simulink model "ECM_EKF_WLTP"  (R2021b)
settings: Solver=FixedStepDiscrete  StartTime=0.0  StopTime=10000  FixedStep=Ts_data  RelTol=1e-3
PreLoadFcn:
  | bdclose all
  | open_system('mdl/ECM_EKF_WLTP')
  | get_param(bdroot,'DataDictionary')
undefined symbols (not defined in the file or in its folder): C1_lut, C2_lut, crate_bp, DiscIntNeverNeededParam, R0_lut, R1_lut, R2_lut, raptor_get_param_eval, raptor_xcp_function, SoC0_guess, soc_bp, Ts_data
libraries: arc_dd_lib x12, Raptor_lib x8, arc_specialized_lib x4, simulink x2, arc_logic_lib x2, arc_fault_lib x2
(part 1 of 2)
settings Model: DataDictionary=ecm_dd.sldd  Creator=ahmeds28  LastModifiedBy=ahmeds28

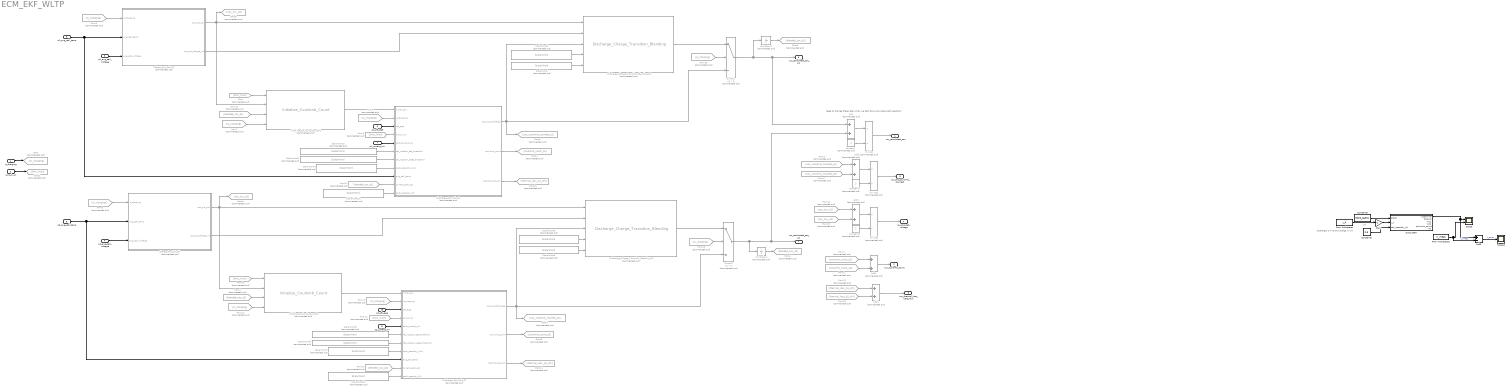
== system ECM_EKF_WLTP ==
  note: Need to change these later when we start allowing single pack operation
  note: discharge is +ve and charge is -ve
  is_charging : Inport  OutDataTypeStr=boolean
  bms_hvon : Inport  Port=2  OutDataTypeStr=boolean
  p1_avg_cell_voltage : Inport  Port=3  OutDataTypeStr=double
  p2_avg_cell_voltage : Inport  Port=4  OutDataTypeStr=double
  p1_avg_cell_temp : Inport  Port=5  OutDataTypeStr=double
  p2_avg_cell_temp : Inport  Port=6  OutDataTypeStr=double
  p1_current_mA : Inport  Port=7  OutDataTypeStr=double
  p2_current_mA : Inport  Port=8  OutDataTypeStr=double
  p1_sfp_age : Inport  Port=9  OutDataTypeStr=uint16
  p2_sfp_age : Inport  Port=10  OutDataTypeStr=uint16
  Add{,1..4} (5 alike) : Sum  Commented=on
  Add5 : Sum  Inputs=+-
  Charge_Soc_Calc_P1 : Subsystem  Commented=on
  Charge_Soc_Calc_P2 : Subsystem  Commented=on
  Constant : Constant  Commented=on  Value=2
  Constant1 : Constant  Commented=on  Value=2
  Constant2 : Constant  Commented=on  Value=2
  Constant3 : Constant  Value=2.5
  Constant5 : Constant  Value=SoC0_guess
  Discharge_Charge_Transition_Blending_P1 : arc_specialized_lib/Discharge_Charge_Transition_Blending  Commented=on  SystemSampleTime=-1  SSRTWFcnClass=[]  VariantActivationTime=update diagram  Latency=0  AutoFrameSizeCalculation=off
  Discharge_Charge_Transition_Blending_P2 : arc_specialized_lib/Discharge_Charge_Transition_Blending  Commented=on  SystemSampleTime=-1  SSRTWFcnClass=[]  VariantActivationTime=update diagram  Latency=0  AutoFrameSizeCalculation=off
  Discharge_Soc_Calc_P1 : Subsystem  Commented=on
  Discharge_Soc_Calc_P2 : Subsystem  Commented=on
  Divide : Product  Commented=on  Inputs=*/
  Divide1 : Product  Commented=on  Inputs=*/
  Divide2 : Product  Commented=on  Inputs=*/
  From{,9..10,12} (4 alike) : From  Commented=on  GotoTag=bms_hvon
  From Workspace : FromWorkspace  VariableName=I_A
  From Workspace1 : FromWorkspace  VariableName=V_meas
  From1 : From  Commented=on  GotoTag=coulomb_count_p1
  From{5..8,11,13,15..16} (8 alike) : From  Commented=on  GotoTag=is_charging
  From14 : From  Commented=on  GotoTag=blended_soc_p1
  From17 : From  Commented=on  GotoTag=soc_coulomb_counted_p2
  From18 : From  Commented=on  GotoTag=soc_ocv_p1
  From19 : From  Commented=on  GotoTag=soc_ocv_p2
  From2 : From  Commented=on  GotoTag=coulomb_count_p2
  From20 : From  Commented=on  GotoTag=blended_soc_p2
  From21 : From  Commented=on  GotoTag=blended_soc_p1
  From22 : From  Commented=on  GotoTag=thermal_loss_p1_Wh
  From23 : From  Commented=on  GotoTag=thermal_loss_p2_Wh
  From3 : From  Commented=on  GotoTag=soc_coulomb_counted_p1
  From4 : From  Commented=on  GotoTag=blended_soc_p2
  Gain : Gain  Gain=-1
  Goto : Goto  Commented=on  GotoTag=is_charging
  Goto1 : Goto  Commented=on  GotoTag=blended_soc_p2
  Goto10 : Goto  Commented=on  GotoTag=thermal_loss_p1_Wh
  Goto11 : Goto  Commented=on  GotoTag=thermal_loss_p2_Wh
  Goto2 : Goto  Commented=on  GotoTag=bms_hvon
  Goto3 : Goto  Commented=on  GotoTag=blended_soc_p1
  Goto4 : Goto  Commented=on  GotoTag=coulomb_count_p1
  Goto5 : Goto  Commented=on  GotoTag=coulomb_count_p2
  Goto6 : Goto  Commented=on  GotoTag=soc_coulomb_counted_p1
  Goto7 : Goto  Commented=on  GotoTag=soc_coulomb_counted_p2
  Goto8 : Goto  Commented=on  GotoTag=soc_ocv_p1
  Goto9 : Goto  Commented=on  GotoTag=soc_ocv_p2
  Initialize_Coulomb_Count_P1 : arc_specialized_lib/Initialize_Coulomb_Count  Commented=on  SystemSampleTime=-1  SSRTWFcnClass=[]  VariantActivationTime=update diagram  Latency=0  AutoFrameSizeCalculation=off
  Initialize_Coulomb_Count_P2 : arc_specialized_lib/Initialize_Coulomb_Count  Commented=on  SystemSampleTime=-1  SSRTWFcnClass=[]  VariantActivationTime=update diagram  Latency=0  AutoFrameSizeCalculation=off
  ScalarWord : arc_dd_lib/DataParam/ScalarWord  Tag=TYPE:UInt8; LSB:0.015625; OFF:0; RANGE:(0,3); UNIT:adm;  Description=Scalar Calibration  Commented=on  ScalarVar_Name=charge_soc_upper_limit  ScalarVar_Value=95  ScalarVar_Min=0  ScalarVar_Max=100  ScalarVar_dType=uint8  ScalarVar_dUnit=%  ScalarVar_dT=inf  ScalarVar_vType=Coefficient (k)  ScalarVar_Description=Insert variable description here.  SSRTWFcnClass=[]
  ScalarWord1 : arc_dd_lib/DataParam/ScalarWord  Tag=TYPE:UInt8; LSB:0.015625; OFF:0; RANGE:(0,3); UNIT:adm;  Description=Scalar Calibration  Commented=on  ScalarVar_Name=blending_distance  ScalarVar_Value=20  ScalarVar_Min=0  ScalarVar_Max=100  ScalarVar_dType=uint8  ScalarVar_dUnit=%  ScalarVar_dT=inf  ScalarVar_vType=Coefficient (k)  ScalarVar_Description=Insert variable description here.  SSRTWFcnClass=[]
  ScalarWord10 : arc_dd_lib/DataParam/ScalarWord  Tag=TYPE:UInt8; LSB:0.015625; OFF:0; RANGE:(0,3); UNIT:adm;  Description=Scalar Calibration  Commented=on  ScalarVar_Name=single_pack_energy_capacity  ScalarVar_Value=110000  ScalarVar_Min=0  ScalarVar_Max=1e7  ScalarVar_dType=uint32  ScalarVar_dUnit=Wh  ScalarVar_dT=inf  ScalarVar_vType=Coefficient (k)  ScalarVar_Description=Insert variable description here.  SSRTWFcnClass=[]
  ScalarWord11 : arc_dd_lib/DataParam/ScalarWord  Tag=TYPE:UInt8; LSB:0.015625; OFF:0; RANGE:(0,3); UNIT:adm;  Description=Scalar Calibration  Commented=on  ScalarVar_Name=single_pack_energy_capacity  ScalarVar_Value=110000  ScalarVar_Min=0  ScalarVar_Max=1e7  ScalarVar_dType=uint32  ScalarVar_dUnit=Wh  ScalarVar_dT=inf  ScalarVar_vType=Coefficient (k)  ScalarVar_Description=Insert variable description here.  SSRTWFcnClass=[]
  ScalarWord2 : arc_dd_lib/DataParam/ScalarWord  Tag=TYPE:UInt8; LSB:0.015625; OFF:0; RANGE:(0,3); UNIT:adm;  Description=Scalar Calibration  Commented=on  ScalarVar_Name=current_sensor_lossCan_set_threshold  ScalarVar_Value=100  ScalarVar_Min=0  ScalarVar_Max=65534  ScalarVar_dType=uint16  ScalarVar_dT=inf  ScalarVar_vType=Coefficient (k)  ScalarVar_Description=Insert variable description here.  SSRTWFcnClass=[]
  ScalarWord3 : arc_dd_lib/DataParam/ScalarWord  Tag=TYPE:UInt8; LSB:0.015625; OFF:0; RANGE:(0,3); UNIT:adm;  Description=Scalar Calibration  Commented=on  ScalarVar_Name=current_sensor_lossCan_reset_threshold  ScalarVar_Value=0  ScalarVar_Min=0  ScalarVar_Max=65534  ScalarVar_dType=uint16  ScalarVar_dT=inf  ScalarVar_vType=Coefficient (k)  ScalarVar_Description=Insert variable description here.  SSRTWFcnClass=[]
  ScalarWord4 : arc_dd_lib/DataParam/ScalarWord  Tag=TYPE:UInt8; LSB:0.015625; OFF:0; RANGE:(0,3); UNIT:adm;  Description=Scalar Calibration  Commented=on  ScalarVar_Name=single_pack_capacity  ScalarVar_Value=160000  ScalarVar_Min=0  ScalarVar_Max=1e7  ScalarVar_dType=uint32  ScalarVar_dUnit=mAh  ScalarVar_dT=inf  ScalarVar_vType=Coefficient (k)  ScalarVar_Description=Insert variable description here.  SSRTWFcnClass=[]
  ScalarWord5 : arc_dd_lib/DataParam/ScalarWord  Tag=TYPE:UInt8; LSB:0.015625; OFF:0; RANGE:(0,3); UNIT:adm;  Description=Scalar Calibration  Commented=on  ScalarVar_Name=current_sensor_lossCan_set_threshold  ScalarVar_Value=100  ScalarVar_Min=0  ScalarVar_Max=65534  ScalarVar_dType=uint16  ScalarVar_dT=inf  ScalarVar_vType=Coefficient (k)  ScalarVar_Description=Insert variable description here.  SSRTWFcnClass=[]
  ScalarWord6 : arc_dd_lib/DataParam/ScalarWord  Tag=TYPE:UInt8; LSB:0.015625; OFF:0; RANGE:(0,3); UNIT:adm;  Description=Scalar Calibration  Commented=on  ScalarVar_Name=current_sensor_lossCan_reset_threshold  ScalarVar_Value=0  ScalarVar_Min=0  ScalarVar_Max=65534  ScalarVar_dType=uint16  ScalarVar_dT=inf  ScalarVar_vType=Coefficient (k)  ScalarVar_Description=Insert variable description here.  SSRTWFcnClass=[]
  ScalarWord7 : arc_dd_lib/DataParam/ScalarWord  Tag=TYPE:UInt8; LSB:0.015625; OFF:0; RANGE:(0,3); UNIT:adm;  Description=Scalar Calibration  Commented=on  ScalarVar_Name=single_pack_capacity  ScalarVar_Value=160000  ScalarVar_Min=0  ScalarVar_Max=1e7  ScalarVar_dType=uint32  ScalarVar_dUnit=mAh  ScalarVar_dT=inf  ScalarVar_vType=Coefficient (k)  ScalarVar_Description=Insert variable description here.  SSRTWFcnClass=[]
  ScalarWord8 : arc_dd_lib/DataParam/ScalarWord  Tag=TYPE:UInt8; LSB:0.015625; OFF:0; RANGE:(0,3); UNIT:adm;  Description=Scalar Calibration  Commented=on  ScalarVar_Name=charge_soc_upper_limit  ScalarVar_Value=95  ScalarVar_Min=0  ScalarVar_Max=100  ScalarVar_dType=uint8  ScalarVar_dUnit=%  ScalarVar_dT=inf  ScalarVar_vType=Coefficient (k)  ScalarVar_Description=Insert variable description here.  SSRTWFcnClass=[]
  ScalarWord9 : arc_dd_lib/DataParam/ScalarWord  Tag=TYPE:UInt8; LSB:0.015625; OFF:0; RANGE:(0,3); UNIT:adm;  Description=Scalar Calibration  Commented=on  ScalarVar_Name=blending_distance  ScalarVar_Value=20  ScalarVar_Min=0  ScalarVar_Max=100  ScalarVar_dType=uint8  ScalarVar_dUnit=%  ScalarVar_dT=inf  ScalarVar_vType=Coefficient (k)  ScalarVar_Description=Insert variable description here.  SSRTWFcnClass=[]
  Scope : Scope  NumInputPorts=2
  Scope1 : Scope
  Subsystem : Subsystem
  Switch1 : Switch  Commented=on  Criteria=u2 > Threshold
  Switch2 : Switch  Commented=on  Criteria=u2 > Threshold
  Unit Delay1 : UnitDelay  Commented=on  SampleTime=-1  HasFrameUpgradeWarning=on
  Unit Delay2 : UnitDelay  Commented=on  SampleTime=-1  HasFrameUpgradeWarning=on
  vcu_calculated_soc : Outport  OutDataTypeStr=double
  vcu_coulomb_count : Outport  Port=2  OutDataTypeStr=single
  vcu_soc_coulomb_counted : Outport  Port=3  OutDataTypeStr=double
  vcu_soc_cell_voltage : Outport  Port=4  OutDataTypeStr=double
  vcu_thermal_loss_watt_hour : Outport  Port=5  OutDataTypeStr=single
  vcu_calculated_soc_p1 : Outport  Port=6  OutDataTypeStr=double
  vcu_calculated_soc_p2 : Outport  Port=7  OutDataTypeStr=double
  wires:
  Switch1/1 -> Unit Delay2/1, Add/1, vcu_calculated_soc_p1/1
  p1_avg_cell_temp/1 -> Discharge_Soc_Calc_P1/9(avg_cell_temp), Charge_Soc_Calc_P1/2(avg_cell_temp)
  From7/1 -> Initialize_Coulomb_Count_P1/4
  is_charging/1 -> Goto/1
  ScalarWord/1 -> Discharge_Charge_Transition_Blending_P1/5
  p1_avg_cell_voltage/1 -> Charge_Soc_Calc_P1/3(avg_cell_voltage)
  Add4/1 -> vcu_thermal_loss_watt_hour/1
  Discharge_Soc_Calc_P1/3(thermal_loss_Wh) -> Goto10/1
  From14/1 -> Initialize_Coulomb_Count_P1/3
  From/1 -> Initialize_Coulomb_Count_P1/1
  Switch2/1 -> Unit Delay1/1, Add/2, vcu_calculated_soc_p2/1
  From3/1 -> Add2/1
  p2_sfp_age/1 -> Discharge_Soc_Calc_P2/3(sfp_age)
  bms_hvon/1 -> Goto2/1
  Divide2/1 -> vcu_soc_cell_voltage/1
  From11/1 -> Initialize_Coulomb_Count_P2/4
  Charge_Soc_Calc_P2/1(soc_out_ocv) -> Goto9/1, Discharge_Charge_Transition_Blending_P2/1, Initialize_Coulomb_Count_P2/2
  Add/1 -> Divide/1
  Charge_Soc_Calc_P1/1(soc_out_ocv) -> Goto8/1, Initialize_Coulomb_Count_P1/2, Discharge_Charge_Transition_Blending_P1/1
  Discharge_Charge_Transition_Blending_P1/1 -> Switch1/1
  Discharge_Soc_Calc_P2/1(soc_out_discharge) -> Goto7/1, Switch2/3, Discharge_Charge_Transition_Blending_P2/3
  From4/1 -> Initialize_Coulomb_Count_P2/3
  Unit Delay1/1 -> Goto1/1
  Add3/1 -> Divide2/1
  Discharge_Soc_Calc_P2/2(coulomb_count) -> Goto5/1
  ScalarWord11/1 -> Discharge_Soc_Calc_P2/11(pack_capacity_Wh)
  Discharge_Soc_Calc_P1/2(coulomb_count) -> Goto4/1
  From2/1 -> Add1/2
  Constant1/1 -> Divide1/2
  Add2/1 -> Divide1/1
  From18/1 -> Add3/1
  ScalarWord1/1 -> Discharge_Charge_Transition_Blending_P1/4
  Add1/1 -> vcu_coulomb_count/1
  From15/1 -> Switch1/2
  p1_sfp_age/1 -> Discharge_Soc_Calc_P1/3(sfp_age)
  From22/1 -> Add4/1
  Constant/1 -> Divide/2
  Unit Delay2/1 -> Goto3/1
  Initialize_Coulomb_Count_P2/1 -> Discharge_Soc_Calc_P2/1(initial_soc)
  Charge_Soc_Calc_P1/2(soc_out_charge_init) -> Discharge_Charge_Transition_Blending_P1/2
  Initialize_Coulomb_Count_P1/1 -> Discharge_Soc_Calc_P1/1(initial_soc)
  ScalarWord3/1 -> Discharge_Soc_Calc_P1/7(sfp_lossCan_reset_threshold)
  Constant2/1 -> Divide2/2
  ScalarWord2/1 -> Discharge_Soc_Calc_P1/6(sfp_lossCan_set_threshold)
  From19/1 -> Add3/2
  From6/1 -> Charge_Soc_Calc_P1/1(is_charging)
  From17/1 -> Add2/2
  ScalarWord10/1 -> Discharge_Soc_Calc_P1/11(pack_capacity_Wh)
  Divide/1 -> vcu_calculated_soc/1
  p2_current_mA/1 -> Discharge_Soc_Calc_P2/5(pack_current_mA)
  Charge_Soc_Calc_P2/2(soc_out_charge_init) -> Discharge_Charge_Transition_Blending_P2/2
  ScalarWord6/1 -> Discharge_Soc_Calc_P2/7(sfp_lossCan_reset_threshold)
  Discharge_Charge_Transition_Blending_P2/1 -> Switch2/1
  ScalarWord8/1 -> Discharge_Charge_Transition_Blending_P2/5
  From8/1 -> Discharge_Soc_Calc_P1/2(is_charging)
  p1_current_mA/1 -> Discharge_Soc_Calc_P1/5(pack_current_mA)
  From10/1 -> Initialize_Coulomb_Count_P2/1
  From20/1 -> Discharge_Soc_Calc_P2/10(current_pack_soc)
  p2_avg_cell_temp/1 -> Discharge_Soc_Calc_P2/9(avg_cell_temp), Charge_Soc_Calc_P2/2(avg_cell_temp)
  ScalarWord4/1 -> Discharge_Soc_Calc_P1/8(pack_capacity_mAh)
  From12/1 -> Discharge_Soc_Calc_P2/4(bms_hvon)
  From9/1 -> Discharge_Soc_Calc_P1/4(bms_hvon)
  From23/1 -> Add4/2
  Discharge_Soc_Calc_P1/1(soc_out_discharge) -> Goto6/1, Switch1/3, Discharge_Charge_Transition_Blending_P1/3
  ScalarWord7/1 -> Discharge_Soc_Calc_P2/8(pack_capacity_mAh)
  ScalarWord9/1 -> Discharge_Charge_Transition_Blending_P2/4
  From16/1 -> Switch2/2
  From13/1 -> Discharge_Soc_Calc_P2/2(is_charging)
  Discharge_Soc_Calc_P2/3(thermal_loss_Wh) -> Goto11/1
  p2_avg_cell_voltage/1 -> Charge_Soc_Calc_P2/3(avg_cell_voltage)
  Divide1/1 -> vcu_soc_coulomb_counted/1
  From21/1 -> Discharge_Soc_Calc_P1/10(current_pack_soc)
  From1/1 -> Add1/1
  ScalarWord5/1 -> Discharge_Soc_Calc_P2/6(sfp_lossCan_set_threshold)
  From5/1 -> Charge_Soc_Calc_P2/1(is_charging)
  Constant3/1 -> Subsystem/3(cell_capacity_Ah)
  From Workspace/1 -> Gain/1  "I_A"
  Constant5/1 -> Subsystem/1(SOC0)
  From Workspace1/1 -> Add5/2, Scope/2  "V_meas"
  Subsystem/1(V_terminal) -> Add5/1, Scope/1
  Gain/1 -> Subsystem/2(I_A)
  Add5/1 -> Scope1/1  "V_error"

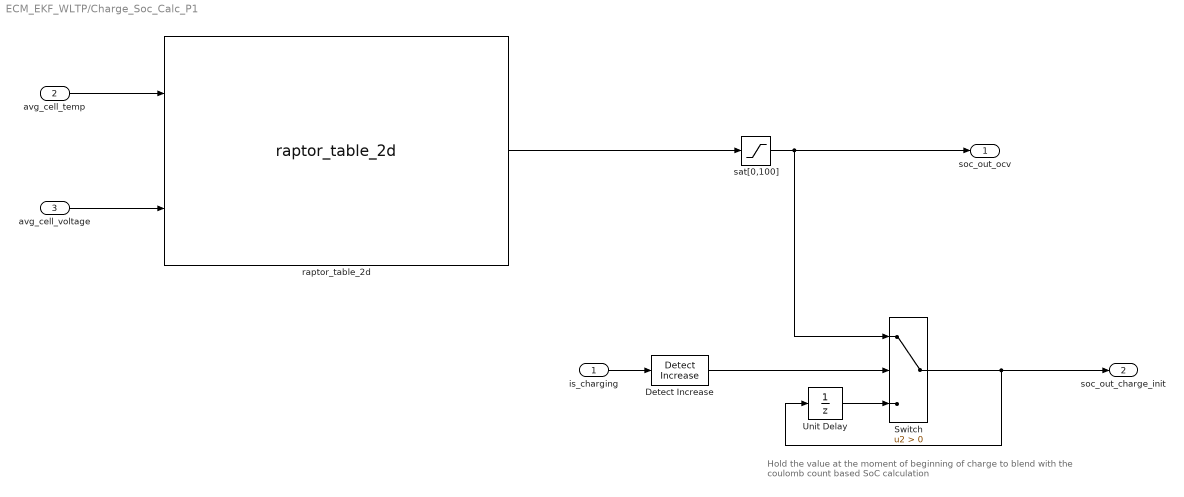
== system ECM_EKF_WLTP/Charge_Soc_Calc_P1 ==
  note: Hold the value at the moment of beginning of charge to blend with the coulomb count based SoC calculation
  is_charging : Inport
  avg_cell_temp : Inport  Port=2
  avg_cell_voltage : Inport  Port=3
  Detect Increase : simulink/Logic and Bit Operations/Detect Increase  vinit=0.0  OutDataTypeStr=boolean
  Switch : Switch  Criteria=u2 > Threshold
  Unit Delay : UnitDelay  SampleTime=-1  HasFrameUpgradeWarning=on
  raptor_table_2d : Raptor_lib/Table Lookup/raptor_table_2d  dataName='ocv_soc_p1'  initValue=|  dataType=double  storage=Volatile (RAM)  initValueX=[3213 3263 3313 3364 3414 3464 3514 3564 3615 3665 3715 3765 3815 3866 3916 3966 4016 4066 4116 4167 4217 4267]  initValueY=[-30 -25 -20 -15 -10 -5 0 5 10 15 20 25 30 35 40 45 50 55]  dataTypeXY=double  storageXY=Volatile (RAM)  calVisible=on  showTable=off  calGain=1.0  calOffset=0.0  calMax=Inf  calMin=-Inf  calFormat='-1'  calUnit=''  calHelp=''  showBreakpointX=off  dataNameX=[]  calGainX=1.0  calOffsetX=0.0  calMaxX=Inf  calMinX=-Inf  calFormatX='-1'  calUnitX=''  calHelpX=''  showBreakpointY=off  dataNameY=[]  calGainY=1.0  calOffsetY=0.0  calMaxY=Inf  calMinY=-Inf  calFormatY='-1'  calUnitY=''  calHelpY=''  calAccess=1  calFunction=raptor_xcp_function(gcb)  measureEnable=off  mName=[raptor_get_param_eval(gcb,'dataName'), '_Output']
      | [0	0	0	0	0	0	0	0	-20.4761904761904	10.6168831168831	21.4115646258503	30.1825396825397	38.2251082251082	45.6994047619047	53.3333333333333	60.7359307359307	68.2422969187676	75.5222734254993	83.6175115207373	91.2675070028011	97.0007680491551	101.048387096774;
      | 0	0	0	0	0	0	-8.29931972789122	3.65079365079369	15.3463203463204	25.4846938775510	34.2939244663383	41.8707482993197	49.2857142857143	56.3161375661376	63.5858585858586	70.8134920634920	77.8639455782314	84.8941798941799	91.0714285714286	95.9297052154195	98.9172335600907	101.904761904762;
      | 0	0	0	0	0	0	0	-20.8333333333333	4.26190476190482	18.8721804511278	29.2416225749559	37.1564625850340	43.9849624060150	50.1845238095238	56.4227642276423	62.5435540069686	68.7559523809524	75.1719576719576	82.2689075630252	89.9404761904762	96.3397901533495	100.593220338983;
      | 0	0	0	0	0	0	0	-13.3333333333333	5.78869047619051	20.8441558441559	31.0180623973727	38.7632275132275	44.9149659863946	50.8495670995671	56.5891472868217	62.6071428571428	68.8809523809524	75.0330687830688	82.1218487394958	89.6392496392497	96.3222789115646	100.803571428571;
      | 0	0	0	0	0	0	0	-5.22222222222217	11.1746031746032	26.5986394557823	36.5262515262515	42.9609279609280	48.8961038961039	54.2162698412698	59.7407407407407	65.6655844155844	71.3690476190477	77.2241579558653	83.4285714285714	90.0884353741497	96.3868003341688	100.789473684211;
      | 0	0	0	0	0	0	0	-20.5555555555554	13.0442176870749	28.3458646616542	37.7128427128427	44.1780045351474	49.4169096209913	54.6329365079365	60.1893939393939	65.8928571428571	71.5963203463204	77.3532668881506	83.3449477351916	89.5773809523810	95.7099567099567	100.272727272727;
      | 0	0	0	0	0	0	0	-6.41025641025635	11.7399267399268	28.5317460317461	38.3189033189033	44.4426406926407	49.8176291793313	55.0529100529100	60.6746031746032	66.5396825396825	72.0263424518744	77.5270562770563	83.3056478405316	89.4523809523810	95.6850459482039	100.087719298246;
      | 0	0	0	0	0	0	-9.48979591836741	2.46031746031750	15.5860805860806	31.7669172932331	41.0859465737515	46.7740429505135	51.6946778711485	56.7162698412698	62.1212121212121	67.7018633540372	72.9640427599612	78.2168186423506	83.7142857142857	89.5975056689343	95.6732348111659	100;
      | 0	0	0	0	0	0	-3.30952380952385	5.06172839506176	17.3299319727892	33.6090225563910	42.6190476190476	48.0860805860806	53.0285714285714	58.3126293995859	63.7681159420290	69.2236024844720	74.4841269841270	79.6161321671525	84.9392097264438	90.6689342403628	96.1904761904762	100.517241379310;
      | 0	0	0	0	0	0	-0.299539170506954	7.70833333333336	19.4322344322345	35.1488095238095	43.7367724867725	48.9514652014652	53.7061994609164	58.7996031746032	64.2962962962963	69.5684523809524	74.6047619047620	79.7181729834791	84.8396501457726	90.3193960511034	95.9841269841270	100.166666666667;
      | 0	0	0	0	0	-1.52691511387166	3.92857142857140	11.1111111111111	21.4136904761905	36.7532467532468	45.5109126984127	50.6223893065998	55.0280112044818	59.9486461251167	65.2721088435374	70.3781512605042	75.3047619047619	80.3174603174604	85.2639751552795	90.7879818594104	96.2550443906376	100.508474576271;
      | 0	0	0	0	-7.87301587301590	0.492063492063456	7.82229965156791	15.2083333333334	24.8809523809524	39.9206349206349	47.9880952380952	53.0442176870748	57.6684636118598	62.5476190476190	67.5163398692810	72.3901098901099	77.1340388007055	81.7813051146385	86.5428571428572	91.6269841269841	96.3492063492064	100.151515151515;
      | 0	0	0	0	-9.51058201058206	4.43121693121687	10.9398496240601	18.2222222222222	26.9799498746867	41.1904761904762	49.9851190476191	54.3943191311612	58.7969924812030	63.6476190476190	68.5256410256410	73.1688311688312	77.7821869488536	82.3852813852814	87.0215633423181	91.9807497467072	96.7309145880575	100.714285714286;
      | 0	0	0	0	-4.87711213517668	3.21812596006141	9.55149501661126	16.8279569892473	25.1455026455027	40.1488095238095	49.0764790764791	54.0828924162258	58.7301587301587	63.7220602526725	68.6217948717949	73.3827493261455	78.0599647266314	82.6580086580087	87.3045822102426	92.2060252672498	96.7279942279942	100.530303030303;
      | 0	0	-2.12342079689019	0.437317784256553	2.99805636540330	6.61064425770305	13.2312925170068	20.3535353535354	28.9047619047619	42.3129251700680	50.8245149911817	55.4469507101086	59.8496240601504	64.5732255166217	69.3081761006289	73.9682539682540	78.4863945578231	82.9676870748299	87.5876010781671	92.5121477162294	97.0814132104455	101.129032258065;
      | 0	0	-0.0224292615596995	1.79606625258799	3.61456176673567	6.61518661518659	12.9235880398671	20.3333333333334	28.2451499118166	41.2987012987013	50.5677655677656	55.3592314118630	59.7619047619048	64.5650183150183	69.3081761006289	73.8961038961039	78.4588744588745	82.9676870748299	87.4935064935065	92.2619047619048	96.7819940476191	100.703125000000;
      | -0.591133004926108	0.645085620455078	1.88130424583626	3.11752287121745	4.35374149659864	8.23680823680821	14.3189368770764	21.7171717171717	29.3217893217893	42.0748299319728	51.0690943043884	55.8702791461412	60.2116402116402	64.8589065255732	69.5061728395062	74.0051020408163	78.5497835497836	83.0033416875522	87.4489795918367	92.2060252672498	96.8102796674225	100.793650793651;
      | 0	1.12032312925170	2.24064625850340	3.36096938775510	4.48129251700680	8.64221364221361	14.6677740863787	21.9892473118280	29.6358543417367	42.6785714285714	51.4026915113872	56.5263605442177	61.0259740259740	65.5996472663139	70.2424242424242	74.8051948051948	79.2899659863946	83.6412151067324	88.1878306878307	93.0018674136321	97.4434035909446	101.557377049180]
      settings: SourceProductName=Raptor
  sat[0,100] : Saturate  UpperLimit=100  LowerLimit=0
  soc_out_ocv : Outport
  soc_out_charge_init : Outport  Port=2
  wires:
  avg_cell_temp/1 -> raptor_table_2d/1
  avg_cell_voltage/1 -> raptor_table_2d/2
  is_charging/1 -> Detect Increase/1
  Switch/1 -> Unit Delay/1, soc_out_charge_init/1
  raptor_table_2d/1 -> sat[0,100]/1
  Detect Increase/1 -> Switch/2
  sat[0,100]/1 -> Switch/1, soc_out_ocv/1
  Unit Delay/1 -> Switch/3

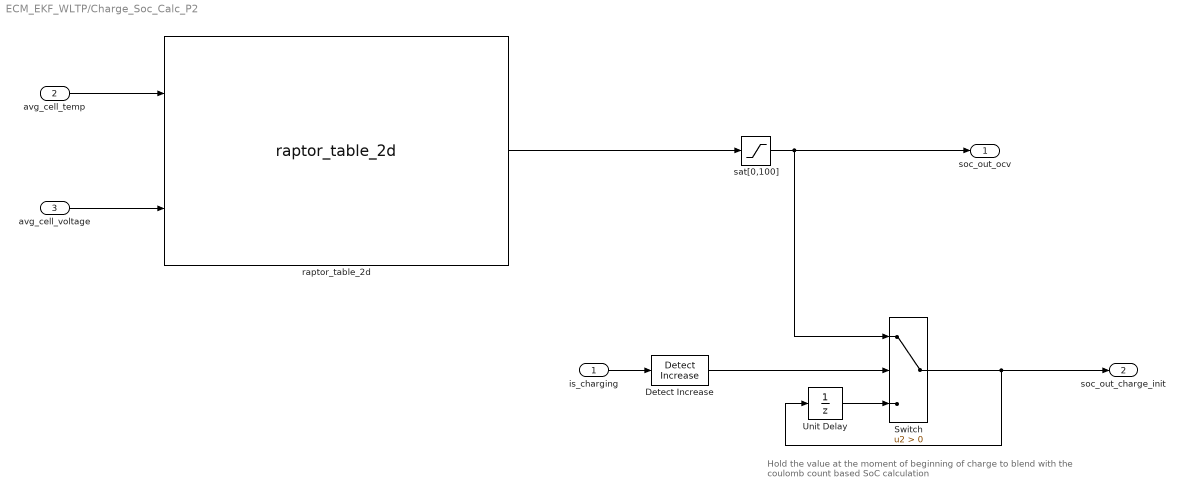
== system ECM_EKF_WLTP/Charge_Soc_Calc_P2 ==
  note: Hold the value at the moment of beginning of charge to blend with the coulomb count based SoC calculation
  is_charging : Inport
  avg_cell_temp : Inport  Port=2
  avg_cell_voltage : Inport  Port=3
  Detect Increase : simulink/Logic and Bit Operations/Detect Increase  vinit=0.0  OutDataTypeStr=boolean
  Switch : Switch  Criteria=u2 > Threshold
  Unit Delay : UnitDelay  SampleTime=-1  HasFrameUpgradeWarning=on
  raptor_table_2d : Raptor_lib/Table Lookup/raptor_table_2d  dataName='ocv_soc_p2'  initValue=|  dataType=double  storage=Volatile (RAM)  initValueX=[3213 3263 3313 3364 3414 3464 3514 3564 3615 3665 3715 3765 3815 3866 3916 3966 4016 4066 4116 4167 4217 4267]  initValueY=[-30 -25 -20 -15 -10 -5 0 5 10 15 20 25 30 35 40 45 50 55]  dataTypeXY=double  storageXY=Volatile (RAM)  calVisible=on  showTable=off  calGain=1.0  calOffset=0.0  calMax=Inf  calMin=-Inf  calFormat='-1'  calUnit=''  calHelp=''  showBreakpointX=off  dataNameX=[]  calGainX=1.0  calOffsetX=0.0  calMaxX=Inf  calMinX=-Inf  calFormatX='-1'  calUnitX=''  calHelpX=''  showBreakpointY=off  dataNameY=[]  calGainY=1.0  calOffsetY=0.0  calMaxY=Inf  calMinY=-Inf  calFormatY='-1'  calUnitY=''  calHelpY=''  calAccess=1  calFunction=raptor_xcp_function(gcb)  measureEnable=off  mName=[raptor_get_param_eval(gcb,'dataName'), '_Output']
      | [0	0	0	0	0	0	0	0	-20.4761904761904	10.6168831168831	21.4115646258503	30.1825396825397	38.2251082251082	45.6994047619047	53.3333333333333	60.7359307359307	68.2422969187676	75.5222734254993	83.6175115207373	91.2675070028011	97.0007680491551	101.048387096774;
      | 0	0	0	0	0	0	-8.29931972789122	3.65079365079369	15.3463203463204	25.4846938775510	34.2939244663383	41.8707482993197	49.2857142857143	56.3161375661376	63.5858585858586	70.8134920634920	77.8639455782314	84.8941798941799	91.0714285714286	95.9297052154195	98.9172335600907	101.904761904762;
      | 0	0	0	0	0	0	0	-20.8333333333333	4.26190476190482	18.8721804511278	29.2416225749559	37.1564625850340	43.9849624060150	50.1845238095238	56.4227642276423	62.5435540069686	68.7559523809524	75.1719576719576	82.2689075630252	89.9404761904762	96.3397901533495	100.593220338983;
      | 0	0	0	0	0	0	0	-13.3333333333333	5.78869047619051	20.8441558441559	31.0180623973727	38.7632275132275	44.9149659863946	50.8495670995671	56.5891472868217	62.6071428571428	68.8809523809524	75.0330687830688	82.1218487394958	89.6392496392497	96.3222789115646	100.803571428571;
      | 0	0	0	0	0	0	0	-5.22222222222217	11.1746031746032	26.5986394557823	36.5262515262515	42.9609279609280	48.8961038961039	54.2162698412698	59.7407407407407	65.6655844155844	71.3690476190477	77.2241579558653	83.4285714285714	90.0884353741497	96.3868003341688	100.789473684211;
      | 0	0	0	0	0	0	0	-20.5555555555554	13.0442176870749	28.3458646616542	37.7128427128427	44.1780045351474	49.4169096209913	54.6329365079365	60.1893939393939	65.8928571428571	71.5963203463204	77.3532668881506	83.3449477351916	89.5773809523810	95.7099567099567	100.272727272727;
      | 0	0	0	0	0	0	0	-6.41025641025635	11.7399267399268	28.5317460317461	38.3189033189033	44.4426406926407	49.8176291793313	55.0529100529100	60.6746031746032	66.5396825396825	72.0263424518744	77.5270562770563	83.3056478405316	89.4523809523810	95.6850459482039	100.087719298246;
      | 0	0	0	0	0	0	-9.48979591836741	2.46031746031750	15.5860805860806	31.7669172932331	41.0859465737515	46.7740429505135	51.6946778711485	56.7162698412698	62.1212121212121	67.7018633540372	72.9640427599612	78.2168186423506	83.7142857142857	89.5975056689343	95.6732348111659	100;
      | 0	0	0	0	0	0	-3.30952380952385	5.06172839506176	17.3299319727892	33.6090225563910	42.6190476190476	48.0860805860806	53.0285714285714	58.3126293995859	63.7681159420290	69.2236024844720	74.4841269841270	79.6161321671525	84.9392097264438	90.6689342403628	96.1904761904762	100.517241379310;
      | 0	0	0	0	0	0	-0.299539170506954	7.70833333333336	19.4322344322345	35.1488095238095	43.7367724867725	48.9514652014652	53.7061994609164	58.7996031746032	64.2962962962963	69.5684523809524	74.6047619047620	79.7181729834791	84.8396501457726	90.3193960511034	95.9841269841270	100.166666666667;
      | 0	0	0	0	0	-1.52691511387166	3.92857142857140	11.1111111111111	21.4136904761905	36.7532467532468	45.5109126984127	50.6223893065998	55.0280112044818	59.9486461251167	65.2721088435374	70.3781512605042	75.3047619047619	80.3174603174604	85.2639751552795	90.7879818594104	96.2550443906376	100.508474576271;
      | 0	0	0	0	-7.87301587301590	0.492063492063456	7.82229965156791	15.2083333333334	24.8809523809524	39.9206349206349	47.9880952380952	53.0442176870748	57.6684636118598	62.5476190476190	67.5163398692810	72.3901098901099	77.1340388007055	81.7813051146385	86.5428571428572	91.6269841269841	96.3492063492064	100.151515151515;
      | 0	0	0	0	-9.51058201058206	4.43121693121687	10.9398496240601	18.2222222222222	26.9799498746867	41.1904761904762	49.9851190476191	54.3943191311612	58.7969924812030	63.6476190476190	68.5256410256410	73.1688311688312	77.7821869488536	82.3852813852814	87.0215633423181	91.9807497467072	96.7309145880575	100.714285714286;
      | 0	0	0	0	-4.87711213517668	3.21812596006141	9.55149501661126	16.8279569892473	25.1455026455027	40.1488095238095	49.0764790764791	54.0828924162258	58.7301587301587	63.7220602526725	68.6217948717949	73.3827493261455	78.0599647266314	82.6580086580087	87.3045822102426	92.2060252672498	96.7279942279942	100.530303030303;
      | 0	0	-2.12342079689019	0.437317784256553	2.99805636540330	6.61064425770305	13.2312925170068	20.3535353535354	28.9047619047619	42.3129251700680	50.8245149911817	55.4469507101086	59.8496240601504	64.5732255166217	69.3081761006289	73.9682539682540	78.4863945578231	82.9676870748299	87.5876010781671	92.5121477162294	97.0814132104455	101.129032258065;
      | 0	0	-0.0224292615596995	1.79606625258799	3.61456176673567	6.61518661518659	12.9235880398671	20.3333333333334	28.2451499118166	41.2987012987013	50.5677655677656	55.3592314118630	59.7619047619048	64.5650183150183	69.3081761006289	73.8961038961039	78.4588744588745	82.9676870748299	87.4935064935065	92.2619047619048	96.7819940476191	100.703125000000;
      | -0.591133004926108	0.645085620455078	1.88130424583626	3.11752287121745	4.35374149659864	8.23680823680821	14.3189368770764	21.7171717171717	29.3217893217893	42.0748299319728	51.0690943043884	55.8702791461412	60.2116402116402	64.8589065255732	69.5061728395062	74.0051020408163	78.5497835497836	83.0033416875522	87.4489795918367	92.2060252672498	96.8102796674225	100.793650793651;
      | 0	1.12032312925170	2.24064625850340	3.36096938775510	4.48129251700680	8.64221364221361	14.6677740863787	21.9892473118280	29.6358543417367	42.6785714285714	51.4026915113872	56.5263605442177	61.0259740259740	65.5996472663139	70.2424242424242	74.8051948051948	79.2899659863946	83.6412151067324	88.1878306878307	93.0018674136321	97.4434035909446	101.557377049180]
      settings: SourceProductName=Raptor
  sat[0,100] : Saturate  UpperLimit=100  LowerLimit=0
  soc_out_ocv : Outport
  soc_out_charge_init : Outport  Port=2
  wires:
  avg_cell_temp/1 -> raptor_table_2d/1
  avg_cell_voltage/1 -> raptor_table_2d/2
  is_charging/1 -> Detect Increase/1
  Switch/1 -> Unit Delay/1, soc_out_charge_init/1
  raptor_table_2d/1 -> sat[0,100]/1
  Detect Increase/1 -> Switch/2
  sat[0,100]/1 -> Switch/1, soc_out_ocv/1
  Unit Delay/1 -> Switch/3

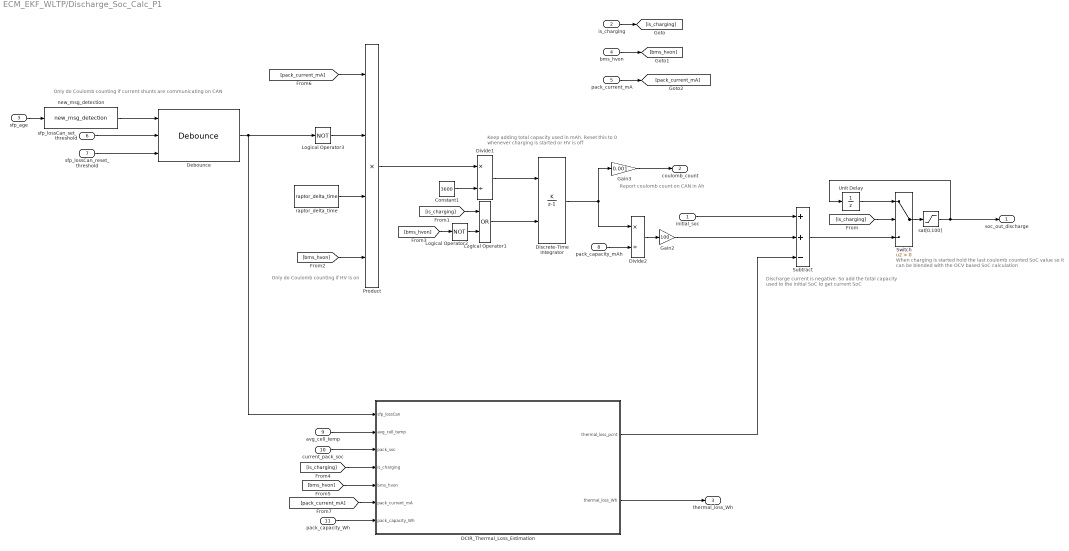
== system ECM_EKF_WLTP/Discharge_Soc_Calc_P1 ==
  note: Only do Coulomb counting if HV is on
  note: Keep adding total capacity used in mAh. Reset this to 0 whenever charging is started or HV is off
  note: Discharge current is negative. So add the total capacity used to the initial SoC to get current SoC
  note: When charging is started hold the last coulomb counted SoC value so it can be blended with the OCV based SoC calculation
  note: Report coulomb count on CAN in Ah
  note: Only do Coulomb counting if current shunts are communicating on CAN
  initial_soc : Inport
  is_charging : Inport  Port=2
  sfp_age : Inport  Port=3
  bms_hvon : Inport  Port=4
  pack_current_mA : Inport  Port=5
  sfp_lossCan_set_threshold : Inport  Port=6
  sfp_lossCan_reset_threshold : Inport  Port=7
  pack_capacity_mAh : Inport  Port=8
  avg_cell_temp : Inport  Port=9
  current_pack_soc : Inport  Port=10
  pack_capacity_Wh : Inport  Port=11
  Constant1 : Constant  Value=3600
  DCIR_Thermal_Loss_Estimation : Subsystem
  Debounce : arc_logic_lib/Debounce  SSRTWFcnClass=[]
  Discrete-Time Integrator : DiscreteIntegrator  IntegratorMethod=Accumulation: Forward Euler  ExternalReset=level  SampleTime=-1  OutDataTypeStr=single  LimitOutput=on  UpperSaturationLimit=175000  LowerSaturationLimit=-175000  ICPrevOutput=DiscIntNeverNeededParam  ICPrevScaledInput=DiscIntNeverNeededParam
      settings: AttributesFormatString=|
      | %<UpperSaturationLimit>
      | %<LowerSaturationLimit>
  Divide1 : Product  Inputs=*/
  Divide2 : Product  Inputs=*/
  Gain2 : Gain  Gain=100
  Gain3 : Gain  Gain=0.001
  Logical Operator1 : Logic  Operator=OR  AllPortsSameDT=off  OutDataTypeStr=boolean
  Logical Operator2 : Logic  Operator=NOT  AllPortsSameDT=off  OutDataTypeStr=boolean
  Logical Operator3 : Logic  Operator=NOT  AllPortsSameDT=off  OutDataTypeStr=boolean
  Product : Product  Inputs=4
  Subtract : Sum  Inputs=++-
  Switch : Switch  Criteria=u2 > Threshold
  Unit Delay : UnitDelay  SampleTime=-1  HasFrameUpgradeWarning=on
  new_msg_detection : arc_fault_lib/new_msg_detection  SystemSampleTime=-1  SSRTWFcnClass=[]  VariantActivationTime=update diagram  Latency=0  AutoFrameSizeCalculation=off
  raptor_delta_time : Raptor_lib/Triggers/raptor_delta_time  unit=seconds
      settings: SourceProductName=Raptor
  sat[0,100] : Saturate  UpperLimit=100  LowerLimit=0
  soc_out_discharge : Outport
  coulomb_count : Outport  Port=2
  thermal_loss_Wh : Outport  Port=3
  wires:
  DCIR_Thermal_Loss_Estimation/1(thermal_loss_pcnt) -> Subtract/3
  DCIR_Thermal_Loss_Estimation/2(thermal_loss_Wh) -> thermal_loss_Wh/1
  pack_capacity_Wh/1 -> DCIR_Thermal_Loss_Estimation/7(pack_capacity_Wh)
  [pack_current_mA] -> DCIR_Thermal_Loss_Estimation/6(pack_current_mA)
  [pack_current_mA] -> Product/1
  [bms_hvon] -> DCIR_Thermal_Loss_Estimation/5(bms_hvon)
  [is_charging] -> DCIR_Thermal_Loss_Estimation/4(is_charging)
  current_pack_soc/1 -> DCIR_Thermal_Loss_Estimation/3(pack_soc)
  avg_cell_temp/1 -> DCIR_Thermal_Loss_Estimation/2(avg_cell_temp)
  [bms_hvon] -> Product/4
  sfp_lossCan_reset_threshold/1 -> Debounce/3
  sfp_lossCan_set_threshold/1 -> Debounce/2
  [bms_hvon] -> Logical Operator2/1
  Logical Operator2/1 -> Logical Operator1/2
  Subtract/1 -> Switch/3
  sat[0,100]/1 -> Unit Delay/1, soc_out_discharge/1
  initial_soc/1 -> Subtract/1
  Switch/1 -> sat[0,100]/1
  [is_charging] -> Switch/2
  [is_charging] -> Logical Operator1/1
  bms_hvon/1 -> [bms_hvon]
  Divide1/1 -> Discrete-Time Integrator/1
  Logical Operator3/1 -> Product/2
  pack_capacity_mAh/1 -> Divide2/2
  Unit Delay/1 -> Switch/1
  sfp_age/1 -> new_msg_detection/1
  Logical Operator1/1 -> Discrete-Time Integrator/2
  Divide2/1 -> Gain2/1
  Discrete-Time Integrator/1 -> Divide2/1, Gain3/1
  pack_current_mA/1 -> [pack_current_mA]
  raptor_delta_time/1 -> Product/3
  new_msg_detection/1 -> Debounce/1
  Constant1/1 -> Divide1/2
  Product/1 -> Divide1/1
  Gain3/1 -> coulomb_count/1
  is_charging/1 -> [is_charging]
  Gain2/1 -> Subtract/2
  Debounce/1 -> DCIR_Thermal_Loss_Estimation/1(sfp_lossCan), Logical Operator3/1

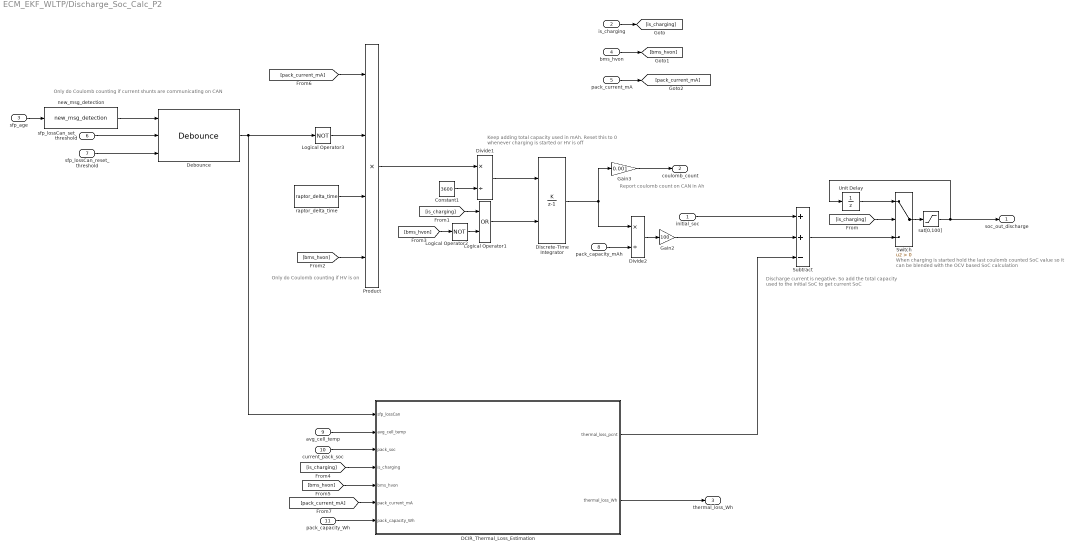
== system ECM_EKF_WLTP/Discharge_Soc_Calc_P2 ==
  note: Only do Coulomb counting if HV is on
  note: Keep adding total capacity used in mAh. Reset this to 0 whenever charging is started or HV is off
  note: Discharge current is negative. So add the total capacity used to the initial SoC to get current SoC
  note: When charging is started hold the last coulomb counted SoC value so it can be blended with the OCV based SoC calculation
  note: Report coulomb count on CAN in Ah
  note: Only do Coulomb counting if current shunts are communicating on CAN
  initial_soc : Inport
  is_charging : Inport  Port=2
  sfp_age : Inport  Port=3
  bms_hvon : Inport  Port=4
  pack_current_mA : Inport  Port=5
  sfp_lossCan_set_threshold : Inport  Port=6
  sfp_lossCan_reset_threshold : Inport  Port=7
  pack_capacity_mAh : Inport  Port=8
  avg_cell_temp : Inport  Port=9
  current_pack_soc : Inport  Port=10
  pack_capacity_Wh : Inport  Port=11
  Constant1 : Constant  Value=3600
  DCIR_Thermal_Loss_Estimation : Subsystem
  Debounce : arc_logic_lib/Debounce
      settings: SourceProductName=Arc Logic Library
  Discrete-Time Integrator : DiscreteIntegrator  IntegratorMethod=Accumulation: Forward Euler  ExternalReset=level  SampleTime=-1  OutDataTypeStr=single  LimitOutput=on  UpperSaturationLimit=175000  LowerSaturationLimit=-175000  ICPrevOutput=DiscIntNeverNeededParam  ICPrevScaledInput=DiscIntNeverNeededParam
      settings: AttributesFormatString=|
      | %<UpperSaturationLimit>
      | %<LowerSaturationLimit>
  Divide1 : Product  Inputs=*/
  Divide2 : Product  Inputs=*/
  Gain2 : Gain  Gain=100
  Gain3 : Gain  Gain=0.001
  Logical Operator1 : Logic  Operator=OR  AllPortsSameDT=off  OutDataTypeStr=boolean
  Logical Operator2 : Logic  Operator=NOT  AllPortsSameDT=off  OutDataTypeStr=boolean
  Logical Operator3 : Logic  Operator=NOT  AllPortsSameDT=off  OutDataTypeStr=boolean
  Product : Product  Inputs=4
  Subtract : Sum  Inputs=++-
  Switch : Switch  Criteria=u2 > Threshold
  Unit Delay : UnitDelay  SampleTime=-1  HasFrameUpgradeWarning=on
  new_msg_detection : arc_fault_lib/new_msg_detection  SystemSampleTime=-1  VariantActivationTime=update diagram  Latency=0  AutoFrameSizeCalculation=off
      settings: SourceProductName=Arc Fault Library
  raptor_delta_time : Raptor_lib/Triggers/raptor_delta_time  unit=seconds
      settings: SourceProductName=Raptor
  sat[0,100] : Saturate  UpperLimit=100  LowerLimit=0
  soc_out_discharge : Outport
  coulomb_count : Outport  Port=2
  thermal_loss_Wh : Outport  Port=3
  wires:
  DCIR_Thermal_Loss_Estimation/1(thermal_loss_pcnt) -> Subtract/3
  DCIR_Thermal_Loss_Estimation/2(thermal_loss_Wh) -> thermal_loss_Wh/1
  pack_capacity_Wh/1 -> DCIR_Thermal_Loss_Estimation/7(pack_capacity_Wh)
  [pack_current_mA] -> DCIR_Thermal_Loss_Estimation/6(pack_current_mA)
  [pack_current_mA] -> Product/1
  [bms_hvon] -> DCIR_Thermal_Loss_Estimation/5(bms_hvon)
  [is_charging] -> DCIR_Thermal_Loss_Estimation/4(is_charging)
  current_pack_soc/1 -> DCIR_Thermal_Loss_Estimation/3(pack_soc)
  avg_cell_temp/1 -> DCIR_Thermal_Loss_Estimation/2(avg_cell_temp)
  [bms_hvon] -> Product/4
  sfp_lossCan_reset_threshold/1 -> Debounce/3
  sfp_lossCan_set_threshold/1 -> Debounce/2
  [bms_hvon] -> Logical Operator2/1
  Logical Operator2/1 -> Logical Operator1/2
  Subtract/1 -> Switch/3
  sat[0,100]/1 -> Unit Delay/1, soc_out_discharge/1
  initial_soc/1 -> Subtract/1
  Switch/1 -> sat[0,100]/1
  [is_charging] -> Switch/2
  [is_charging] -> Logical Operator1/1
  bms_hvon/1 -> [bms_hvon]
  Divide1/1 -> Discrete-Time Integrator/1
  Logical Operator3/1 -> Product/2
  pack_capacity_mAh/1 -> Divide2/2
  Unit Delay/1 -> Switch/1
  sfp_age/1 -> new_msg_detection/1
  Logical Operator1/1 -> Discrete-Time Integrator/2
  Divide2/1 -> Gain2/1
  Discrete-Time Integrator/1 -> Divide2/1, Gain3/1
  pack_current_mA/1 -> [pack_current_mA]
  raptor_delta_time/1 -> Product/3
  new_msg_detection/1 -> Debounce/1
  Constant1/1 -> Divide1/2
  Product/1 -> Divide1/1
  Gain3/1 -> coulomb_count/1
  is_charging/1 -> [is_charging]
  Gain2/1 -> Subtract/2
  Debounce/1 -> DCIR_Thermal_Loss_Estimation/1(sfp_lossCan), Logical Operator3/1

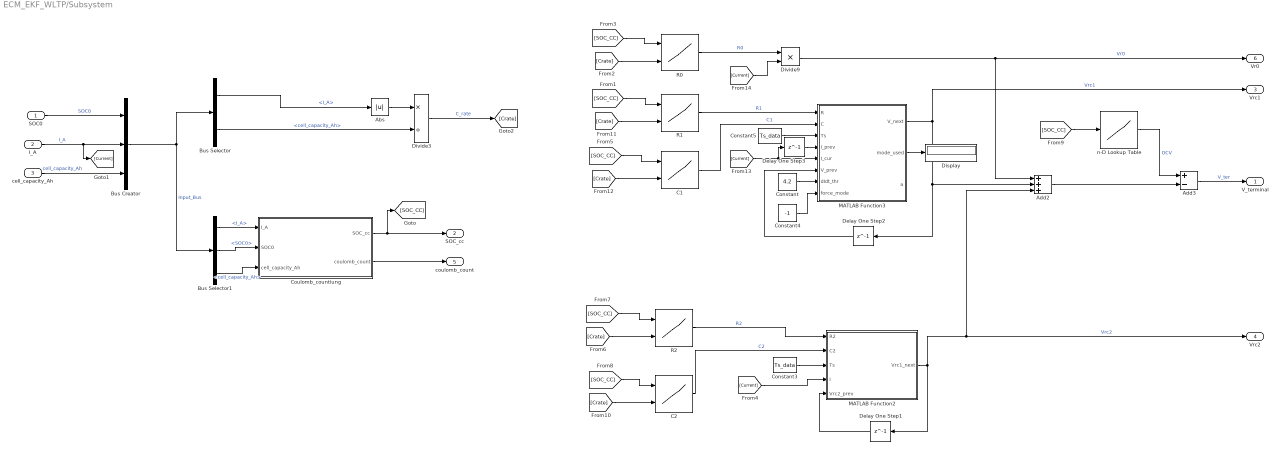
== system ECM_EKF_WLTP/Subsystem ==
  SOC0 : Inport
  I_A : Inport  Port=2
  cell_capacity_Ah : Inport  Port=3
  Abs : Abs
  Add2 : Sum  Inputs=+++
  Add3 : Sum  Inputs=+-
  Bus Creator : BusCreator  Inputs=3
  Bus Selector : BusSelector  OutputSignals=I_A,cell_capacity_Ah
  Bus Selector1 : BusSelector  OutputSignals=I_A,SOC0,cell_capacity_Ah
  C1 : Lookup_n-D  LookupTableObject=''  BreakpointsForDimension1=soc_bp  BreakpointsForDimension2=crate_bp  BreakpointsForDimension3=[5, 7]  BreakpointsForDimension1FirstPoint=10  BreakpointsForDimension2FirstPoint=10  BreakpointsForDimension1Spacing=12  BreakpointsForDimension2Spacing=12  IndexSearchMethod=Linear search  Table=C1_lut  InterpMethod=Flat  DiagnosticForOutOfRangeInput=Error  InternalRulePriority=Speed  RndMeth=Simplest  InputSameDT=on
      settings: InputPortMap=u0,u1
  C2 : Lookup_n-D  LookupTableObject=''  BreakpointsForDimension1=soc_bp  BreakpointsForDimension2=crate_bp  BreakpointsForDimension3=[5, 7]  BreakpointsForDimension1FirstPoint=10  BreakpointsForDimension2FirstPoint=10  BreakpointsForDimension1Spacing=12  BreakpointsForDimension2Spacing=12  IndexSearchMethod=Linear search  Table=C2_lut  InterpMethod=Flat  DiagnosticForOutOfRangeInput=Error  InternalRulePriority=Speed  RndMeth=Simplest  InputSameDT=on
      settings: InputPortMap=u0,u1
  Constant : Constant  Value=4.2
  Constant3 : Constant  Value=Ts_data
  Constant4 : Constant  Value=-1
  Constant5 : Constant  Value=Ts_data
  Coulomb_countiung : Subsystem
  Delay One Step1 : Delay  DelayLength=1
  Delay One Step2 : Delay  DelayLength=1
  Delay One Step3 : Delay  DelayLength=1
  Display : Display
  Divide3 : Product  Inputs=*/
  Divide9 : Product  Inputs=**
  MATLAB Function2 : MATLAB Function  TreatAsAtomicUnit=on
  MATLAB Function3 : MATLAB Function  TreatAsAtomicUnit=on
  R0 : Lookup_n-D  LookupTableObject=''  BreakpointsForDimension1=soc_bp  BreakpointsForDimension2=crate_bp  BreakpointsForDimension3=[5, 7]  BreakpointsForDimension1FirstPoint=10  BreakpointsForDimension2FirstPoint=10  BreakpointsForDimension1Spacing=12  BreakpointsForDimension2Spacing=12  IndexSearchMethod=Linear search  Table=R0_lut  InterpMethod=Flat  DiagnosticForOutOfRangeInput=Error  InternalRulePriority=Speed  RndMeth=Simplest  InputSameDT=on
      settings: InputPortMap=u0,u1
  R1 : Lookup_n-D  LookupTableObject=''  BreakpointsForDimension1=soc_bp  BreakpointsForDimension2=crate_bp  BreakpointsForDimension3=[5, 7]  BreakpointsForDimension1FirstPoint=10  BreakpointsForDimension2FirstPoint=10  BreakpointsForDimension1Spacing=12  BreakpointsForDimension2Spacing=12  IndexSearchMethod=Linear search  Table=R1_lut  InterpMethod=Flat  DiagnosticForOutOfRangeInput=Error  InternalRulePriority=Speed  RndMeth=Simplest  InputSameDT=on
      settings: InputPortMap=u0,u1
  R2 : Lookup_n-D  LookupTableObject=''  BreakpointsForDimension1=soc_bp  BreakpointsForDimension2=crate_bp  BreakpointsForDimension3=[5, 7]  BreakpointsForDimension1FirstPoint=10  BreakpointsForDimension2FirstPoint=10  BreakpointsForDimension1Spacing=12  BreakpointsForDimension2Spacing=12  IndexSearchMethod=Linear search  Table=R2_lut  InterpMethod=Flat  DiagnosticForOutOfRangeInput=Error  InternalRulePriority=Speed  RndMeth=Simplest  InputSameDT=on
      settings: InputPortMap=u0,u1
  n-D Lookup Table : Lookup_n-D  NumberOfTableDimensions=1  BreakpointsForDimension1=[2.5,5,10,15,20,30,40,50,60,70,80,90,95,100]  BreakpointsForDimension3=[5, 7]  Table=[3.077,3.1749,3.1967,3.2132,3.2338,3.2636,3.2838,3.286,3.2892,3.3039,3.3274,3.3292,3.3316,3.4469]  InternalRulePriority=Speed  RndMeth=Simplest  InputSameDT=on
  V_terminal : Outport
  SOC_cc : Outport  Port=2
  Vrc1 : Outport  Port=3
  Vrc2 : Outport  Port=4
  coulomb_count : Outport  Port=5
  Vr0 : Outport  Port=6
  wires:
  Bus Selector/1 -> Abs/1  "<I_A>"
  Bus Selector/2 -> Divide3/2  "<cell_capacity_Ah>"
  Divide3/1 -> [Crate]  "C_rate"
  Abs/1 -> Divide3/1
  [Crate] -> R0/2
  [SOC_CC] -> R0/1
  [Crate] -> R2/2
  [SOC_CC] -> R2/1
  [Crate] -> C2/2
  [SOC_CC] -> C2/1
  R0/1 -> Divide9/1  "R0"
  [Current] -> Divide9/2
  Divide9/1 -> Vr0/1, Add2/1  "Vr0"
  [SOC_CC] -> n-D Lookup Table/1
  n-D Lookup Table/1 -> Add3/1  "OCV"
  Add2/1 -> Add3/2
  Add3/1 -> V_terminal/1  "V_ter"
  [Crate] -> R1/2
  [SOC_CC] -> C1/1
  [Crate] -> C1/2
  R1/1 -> MATLAB Function3/1(R)  "R1"
  C1/1 -> MATLAB Function3/2(C)  "C1"
  [SOC_CC] -> R1/1
  [Current] -> Delay One Step3/1, MATLAB Function3/5(I_cur)
  MATLAB Function3/1(V_next) -> Add2/2, Delay One Step2/1, Vrc1/1  "Vrc1"
  Constant5/1 -> MATLAB Function3/3(Ts)
  Delay One Step1/1 -> MATLAB Function2/5(Vrc2_prev)
  [Current] -> MATLAB Function2/4(I)
  MATLAB Function2/1(Vrc1_next) -> Vrc2/1, Add2/3, Delay One Step1/1  "Vrc2"
  C2/1 -> MATLAB Function2/2(C2)  "C2"
  Constant3/1 -> MATLAB Function2/3(Ts)
  R2/1 -> MATLAB Function2/1(R2)  "R2"
  Delay One Step2/1 -> MATLAB Function3/6(V_prev)
  Delay One Step3/1 -> MATLAB Function3/4(I_prev)
  MATLAB Function3/2(mode_used) -> Display/1
  Constant/1 -> MATLAB Function3/7(dIdt_thr)
  Constant4/1 -> MATLAB Function3/8(force_mode)
  I_A/1 -> [Current], Bus Creator/2  "I_A"
  SOC0/1 -> Bus Creator/1  "SOC0"
  cell_capacity_Ah/1 -> Bus Creator/3  "cell_capacity_Ah"
  Coulomb_countiung/1(SOC_cc) -> [SOC_CC], SOC_cc/1
  Coulomb_countiung/2(coulomb_count) -> coulomb_count/1
  Bus Creator/1 -> Bus Selector1/1, Bus Selector/1  "Input_Bus"
  Bus Selector1/1 -> Coulomb_countiung/1(I_A)  "<I_A>"
  Bus Selector1/3 -> Coulomb_countiung/3(cell_capacity_Ah)  "<cell_capacity_Ah>"
  Bus Selector1/2 -> Coulomb_countiung/2(SOC0)  "<SOC0>"

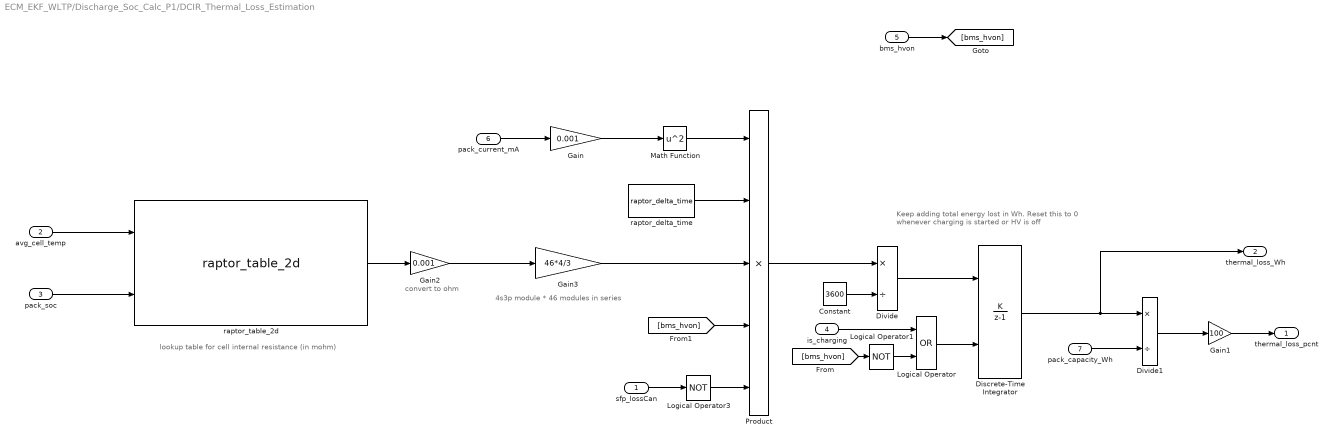
== system ECM_EKF_WLTP/Discharge_Soc_Calc_P1/DCIR_Thermal_Loss_Estimation ==
  note: 4s3p module * 46 modules in series
  note: convert to ohm
  note: lookup table for cell internal resistance (in mohm)
  note: Keep adding total energy lost in Wh. Reset this to 0 whenever charging is started or HV is off
  sfp_lossCan : Inport
  avg_cell_temp : Inport  Port=2
  pack_soc : Inport  Port=3
  is_charging : Inport  Port=4
  bms_hvon : Inport  Port=5
  pack_current_mA : Inport  Port=6
  pack_capacity_Wh : Inport  Port=7
  Constant : Constant  Value=3600
  Discrete-Time Integrator : DiscreteIntegrator  IntegratorMethod=Accumulation: Forward Euler  ExternalReset=level  SampleTime=-1  OutDataTypeStr=single  LimitOutput=on  UpperSaturationLimit=120000  LowerSaturationLimit=0  ICPrevOutput=DiscIntNeverNeededParam  ICPrevScaledInput=DiscIntNeverNeededParam
      settings: AttributesFormatString=|
      | %<UpperSaturationLimit>
      | %<LowerSaturationLimit>
  Divide : Product  Inputs=*/
  Divide1 : Product  Inputs=*/
  Gain : Gain  Gain=0.001
  Gain1 : Gain  Gain=100
  Gain2 : Gain  Gain=0.001
  Gain3 : Gain  Gain=46*4/3
  Logical Operator : Logic  Operator=OR  AllPortsSameDT=off  OutDataTypeStr=boolean
  Logical Operator1 : Logic  Operator=NOT  AllPortsSameDT=off  OutDataTypeStr=boolean
  Logical Operator3 : Logic  Operator=NOT  AllPortsSameDT=off  OutDataTypeStr=boolean
  Math Function : Math  Operator=square  SaturateOnIntegerOverflow=on
  Product : Product  Inputs=5
  raptor_delta_time : Raptor_lib/Triggers/raptor_delta_time  unit=seconds
      settings: SourceProductName=Raptor
  raptor_table_2d : Raptor_lib/Table Lookup/raptor_table_2d  dataName='dcir_p1'  initValue=|  dataType=double  storage=Calibration  initValueX=[5 10 15 20 25 30 35 40 45 50 55 60 65 70 75 80 85 90 95 100]  initValueY=[0 10 25 45]  dataTypeXY=double  storageXY=Calibration  calVisible=on  showTable=off  calGain=1.0  calOffset=0.0  calMax=Inf  calMin=-Inf  calFormat='-1'  calUnit=''  calHelp=''  showBreakpointX=off  dataNameX=[]  calGainX=1.0  calOffsetX=0.0  calMaxX=Inf  calMinX=-Inf  calFormatX='-1'  calUnitX=''  calHelpX=''  showBreakpointY=off  dataNameY=[]  calGainY=1.0  calOffsetY=0.0  calMaxY=Inf  calMinY=-Inf  calFormatY='-1'  calUnitY=''  calHelpY=''  calAccess=1  calFunction=raptor_xcp_function(gcb)  measureEnable=off  mName=[raptor_get_param_eval(gcb,'dataName'), '_Output']
      | [5.77000000000000	5.16400000000000	4.79100000000000	4.55700000000000	4.41700000000000	3.92700000000000	3.85800000000000	3.82300000000000	3.47000000000000	3.46700000000000	3.47200000000000	3.47900000000000	3.48400000000000	3.48600000000000	3.49400000000000	3.51100000000000	3.54500000000000	3.60100000000000	3.73100000000000	4.16700000000000;
      | 2.54900000000000	2.36200000000000	2.27500000000000	2.50700000000000	2.44900000000000	2.31500000000000	2.25000000000000	2.18000000000000	2.18500000000000	2.20700000000000	2.23300000000000	2.24600000000000	2.24200000000000	2.24000000000000	2.24800000000000	2.25000000000000	2.26100000000000	2.28500000000000	2.35800000000000	2.64100000000000;
      | 1.86600000000000	1.67500000000000	1.55200000000000	1.48700000000000	1.42900000000000	1.39400000000000	1.37700000000000	1.35600000000000	1.36400000000000	1.40000000000000	1.44500000000000	1.46200000000000	1.47000000000000	1.46800000000000	1.46100000000000	1.46800000000000	1.47100000000000	1.46800000000000	1.49800000000000	1.68000000000000;
      | 1.27500000000000	1.07800000000000	0.994000000000000	0.934000000000000	0.911000000000000	0.891000000000000	0.880000000000000	0.879000000000000	0.870000000000000	0.877000000000000	0.940000000000000	0.967000000000000	0.967000000000000	0.955000000000000	0.959000000000000	0.958000000000000	0.942000000000000	0.921000000000000	0.920000000000000	1.05600000000000]
      settings: SourceProductName=Raptor
  thermal_loss_pcnt : Outport
  thermal_loss_Wh : Outport  Port=2
  wires:
  pack_current_mA/1 -> Gain/1
  Math Function/1 -> Product/1
  raptor_delta_time/1 -> Product/2
  avg_cell_temp/1 -> raptor_table_2d/1
  pack_soc/1 -> raptor_table_2d/2
  raptor_table_2d/1 -> Gain2/1
  Gain/1 -> Math Function/1
  Product/1 -> Divide/1
  Constant/1 -> Divide/2
  Divide/1 -> Discrete-Time Integrator/1
  Logical Operator/1 -> Discrete-Time Integrator/2
  is_charging/1 -> Logical Operator/1
  Logical Operator1/1 -> Logical Operator/2
  bms_hvon/1 -> [bms_hvon]
  Discrete-Time Integrator/1 -> thermal_loss_Wh/1, Divide1/1
  pack_capacity_Wh/1 -> Divide1/2
  Divide1/1 -> Gain1/1
  Gain1/1 -> thermal_loss_pcnt/1
  [bms_hvon] -> Logical Operator1/1
  [bms_hvon] -> Product/4
  Logical Operator3/1 -> Product/5
  sfp_lossCan/1 -> Logical Operator3/1
  Gain2/1 -> Gain3/1
  Gain3/1 -> Product/3
